simulink model "Linear_with_song_new"  (R2015a)
settings: Solver=ode45  StartTime=0.0  StopTime=30  RelTol=1e-3
libraries: dspvision x2, dspsnks4 x1
settings Model: Creator=ekulasek  LastModifiedBy=ekulasek

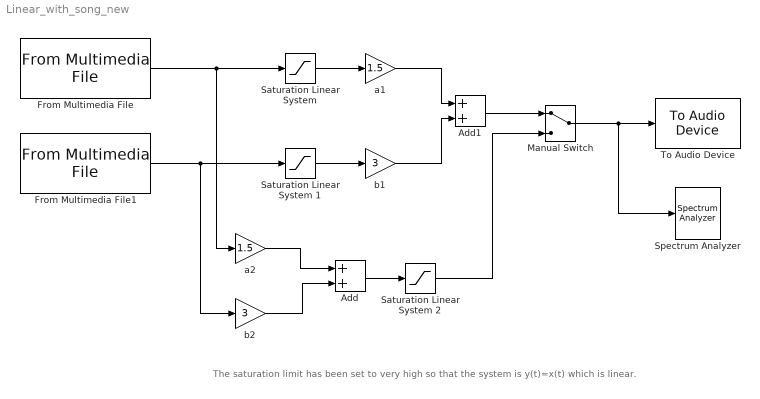
== system Linear_with_song_new ==
  note: The saturation limit has been set to very high so that the system is y(t)=x(t) which is linear.
  Add : Sum
  Add1 : Sum
  From Multimedia File : dspvision/From Multimedia File  inputFilename=/home/ekulasek/Malabe/classes/SignalsAndSystems/Programs/acappeller.wav  loop=on  numPlays=inf  outputStreams=Audio only  videoDataType=single  audioDataType=double  inheritSampleTime=on  userDefinedSampleTime=1/30  noAudioOutput=off  isIntensityVideo=off  fourcc=RGB  colorVideoFormat=Separate color signals  outputEOF=off  dataOrg=Column-major  audioFrameSize=1024  computeAudioFrameSize=off  outSamplingMode=Sample based
  From Multimedia File1 : dspvision/From Multimedia File  inputFilename=/home/ekulasek/Malabe/classes/SignalsAndSystems/Programs/instrumental.wav  loop=on  numPlays=inf  outputStreams=Audio only  videoDataType=single  audioDataType=double  inheritSampleTime=on  userDefinedSampleTime=1/30  noAudioOutput=off  isIntensityVideo=off  fourcc=RGB  colorVideoFormat=Separate color signals  outputEOF=off  dataOrg=Column-major  audioFrameSize=1024  computeAudioFrameSize=off  outSamplingMode=Sample based
  Manual Switch : ManualSwitch
  Saturation Linear System : Saturate  UpperLimit=5  LowerLimit=-5
  Saturation Linear System 1 : Saturate  UpperLimit=5  LowerLimit=-5
  Saturation Linear System 2 : Saturate  UpperLimit=5  LowerLimit=-5
  Spectrum Analyzer : SpectrumAnalyzer
  To Audio Device : dspsnks4/To Audio Device  deviceName=Default  inheritSampleRate=on  sampleRate=44100  deviceDatatype=Determine from input data type  autoBufferSize=on  bufferSize=4096  queueDuration=1.0  defaultOutputChannelMapping=on  outputChannelMapping=1:2  outputNumUnderrunSamples=off
  a1 : Gain  Gain=1.5
  a2 : Gain  Gain=1.5
  b1 : Gain  Gain=3
  b2 : Gain  Gain=3
  wires:
  From Multimedia File1/1 -> b2/1, Saturation Linear System 1/1
  Manual Switch/1 -> Spectrum Analyzer/1, To Audio Device/1
  Add/1 -> Saturation Linear System 2/1
  Saturation Linear System/1 -> a1/1
  Saturation Linear System 1/1 -> b1/1
  Saturation Linear System 2/1 -> Manual Switch/2
  From Multimedia File/1 -> Saturation Linear System/1, a2/1
  a2/1 -> Add/1
  b2/1 -> Add/2
  a1/1 -> Add1/1
  b1/1 -> Add1/2
  Add1/1 -> Manual Switch/1
